simulink model "Plate_aerator"  (Simulink 7.9)
settings: Solver=ode15s  SolverMode=SingleTasking  StartTime=0.0  StopTime=24*3600  MaxStep=1000  RelTol=1e-5  AbsTol=1e-5
undefined symbols (not defined in the file): B, U, x0
settings Model: Creator=psross  LastModifiedBy=M.Sparnaaij  ExtModeTrigMode=oneshot  ExtModeArmWhenConnect=off
settings DataIOCC: LimitDataPoints=off  SaveOutput=off  SaveTime=off  SignalLoggingName=sigsOut
settings OptimizationCC: BooleanDataType=off
settings DebuggingCC: SaveWithParameterizedLinksMsg=none  SignalResolutionControl=TryResolveAllWithWarning  SolverPrmCheckMsg=none  MultiTaskDSMMsg=warning  MultiTaskCondExecSysMsg=none  FcnCallInpInsideContextMsg=Use local settings  StrictBusMsg=None
settings HardwareCC: TargetUnknown=on
settings RTWCC: IncludeERTFirstTime=on
settings GRTTargetCC: CombineOutputUpdateFcns=off  GRTInterface=on

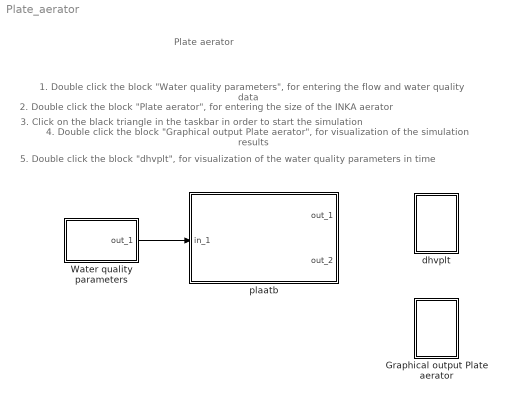
== system Plate_aerator ==
  note: Plate aerator
  note: 2. Double click the block "Plate aerator", for entering the size of the INKA aerator
  note: 3. Click on the black triangle in the taskbar in order to start the simulation
  note: 4. Double click the block "Graphical output Plate aerator", for visualization of the simulation results
  note: 1. Double click the block "Water quality parameters", for entering the flow and water quality data
  note: 5. Double click the block "dhvplt", for visualization of the water quality parameters in time
  Graphical output Plate aerator : Subsystem
      settings: OpenFcn=plaatb_g
      mask Display:
      | plot(0,0,100,100,[80,20,20],[20,20,80],[80,69,60,52,45,39,33,28,24,20],[65,65,64,61,57,52,45,37,30,20])
      | disp('');
      | text(100,100,'plaatb', 'horizontalAlignment', 'right', 'verticalAlignment', 'top');
  Water quality parameters : Subsystem  Description=The water flow and the water quality data must be filled out in the 'Water quality parameters' block. Each project must start with a 'Water quality parameters' block.
      mask init:
      | filenaam='./StimelaData/Water_qual_param.mat';
      | 
      | [Pn,Fn,Fext]=Fileprop(filenaam);
      | 
      | errstr = st_UniqName(filenaam,'filenaam=''','SubSystem','OpenFcn');
      | if errstr, error([errstr 'The filename "' filenaam '" is already in use. Choose a different filename.']), end
      | 
      | P = invruw_p(filenaam);
      | [B,x0,U]=invruw_i(filenaam);
      settings: OpenFcn=|
      | filenaam='./StimelaData/Water_qual_param.mat';
      | st_ParameterInput('init',gcb,filenaam,'invruw');
      mask Display:
      | plot(0,0,100,100,[80 100],[ 50 50],[80 100],[ 55 55],[20 80 80 20 20],[10 10 90  90 10]);
      | disp('')
      | text(50,50,'invruw', 'horizontalAlignment', 'center', 'verticalAlignment', 'middle');
      | text(50,0,Fn, 'horizontalAlignment', 'center', 'verticalAlignment', 'base');
  dhvplt : Subsystem
      settings: OpenFcn=plotStimela2
      mask Display:
      | plot(0,0,100,100,[80,20,20],[20,20,80],[80,69,60,52,45,39,33,28,24,20],[65,65,64,61,57,52,45,37,30,20])
      | disp('');
      | text(100,100,'Stimela', 'horizontalAlignment', 'right', 'verticalAlignment', 'top');
  plaatb : Subsystem  Description=This model calculates the aeration and degassifying with a weir aerator. The influent carbon dioxide concentration is calculated on the basis of the bicarbonate concentration, the pH, the EGV and the water temperature, so these parameters must always be filled out in the 'Water quality parameters' block.
      mask init:
      | filenaam='./StimelaData/Plate_aerator.mat';
      | 
      | [Pn,Fn,Fext]=Fileprop(filenaam);
      | 
      | errstr = st_UniqName(filenaam,'filenaam=''','SubSystem','OpenFcn');
      | if errstr, error([errstr 'The filename "' filenaam '" is already in use. Choose a different filename.']), end
      | 
      | P = plaatb_p(filenaam);
      | [B,x0,U]=plaatb_i(filenaam);
      settings: OpenFcn=|
      | filenaam='./StimelaData/Plate_aerator.mat';
      | st_ParameterInput('init',gcb,filenaam,'plaatb');
      mask Display:
      | plot(0,0,100,100,[20,80,80,20,20],[70,70,20,20,70],[80,90,90,90,9,9,20],[20,20,30,40,40,60,60],[80,20],[50,50],[11,10,8,6],[60,65,68,70],[15,14,12,10,6],[60,64,67,69,70],[78,78],[40,50],[84,83,82,80],[40,45,48,50],[87,86,84,80],[40,45,48,50],[64,64,67,67],[80,77,77,70],[64,73,73,70,70],[80,80,77,77,70],[70,67],[77,77])
      | disp('')
      | text(50,50,'plaatb', 'horizontalAlignment', 'center', 'verticalAlignment', 'middle');
      | text(50,0,Fn, 'horizontalAlignment', 'center', 'verticalAlignment', 'base');
  wires:
  Water quality parameters/1(out_1) -> plaatb/1(in_1)

== system Plate_aerator/Graphical output Plate aerator ==
  note: plotten

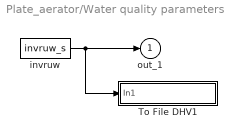
== system Plate_aerator/Water quality parameters ==
  To File DHV1 : Subsystem  mask(To File DHV){naam=[filenaam(1:length(filenaam)-4) '_out.sti']}
      mask prompts: naam "Naam van bestand"
      mask init:
      | set_param([gcb '/To File'],'Filename',naam);
      mask Display: disp(naam)
  invruw : S-Function  FunctionName=invruw_s  Parameters=B,x0,U,P  EnableBusSupport=off
  out_1 : Outport  InitialOutput=0
  wires:
  invruw/1 -> out_1/1, To File DHV1/1(In1)

== system Plate_aerator/dhvplt ==
  note: plotten

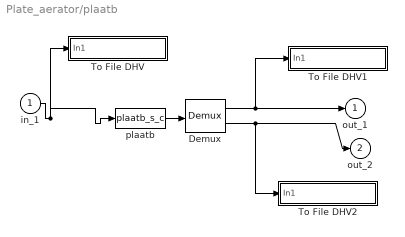
== system Plate_aerator/plaatb ==
  in_1 : Inport
  Demux : Demux  Outputs=[U.Number B.Measurements]
  To File DHV : Subsystem  mask(To File DHV){naam=[filenaam(1:length(filenaam)-4) '_in.sti']}
      mask prompts: naam "Naam van bestand"
      mask init:
      | set_param([gcb '/To File'],'Filename',naam);
      mask Display: disp(naam)
  To File DHV1 : Subsystem  mask(To File DHV){naam=[filenaam(1:length(filenaam)-4) '_out.sti']}
      mask prompts: naam "Naam van bestand"
      mask init:
      | set_param([gcb '/To File'],'Filename',naam);
      mask Display: disp(naam)
  To File DHV2 : Subsystem  mask(To File DHV){naam=[filenaam(1:length(filenaam)-4) '_EM.sti']}
      mask prompts: naam "Naam van bestand"
      mask init:
      | set_param([gcb '/To File'],'Filename',naam);
      mask Display: disp(naam)
  plaatb : S-Function  FunctionName=plaatb_s_c  Parameters=B,x0,U,P  EnableBusSupport=off
  out_1 : Outport  InitialOutput=0
  out_2 : Outport  Port=2  InitialOutput=0
  wires:
  plaatb/1 -> Demux/1
  Demux/1 -> out_1/1, To File DHV1/1(In1)
  Demux/2 -> out_2/1, To File DHV2/1(In1)
  in_1/1 -> plaatb/1, To File DHV/1(In1)

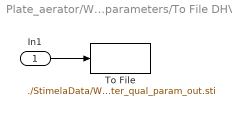
== system Plate_aerator/Water quality parameters/To File DHV1 ==
  In1 : Inport
  To File : ToFile  Filename=./StimelaData/Water_qual_param_out.sti  MatrixName=invruwout
  wires:
  In1/1 -> To File/1

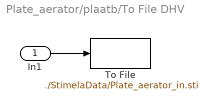
== system Plate_aerator/plaatb/To File DHV ==
  In1 : Inport
  To File : ToFile  Filename=./StimelaData/Plate_aerator_in.sti  MatrixName=plaatbin
  wires:
  In1/1 -> To File/1

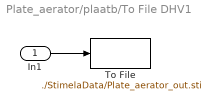
== system Plate_aerator/plaatb/To File DHV1 ==
  In1 : Inport
  To File : ToFile  Filename=./StimelaData/Plate_aerator_out.sti  MatrixName=plaatbout
  wires:
  In1/1 -> To File/1

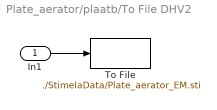
== system Plate_aerator/plaatb/To File DHV2 ==
  In1 : Inport
  To File : ToFile  Filename=./StimelaData/Plate_aerator_EM.sti  MatrixName=plaatbEM
  wires:
  In1/1 -> To File/1
